simulink model "HX_Simulink_Model"  (R2024a)
settings: Solver=FixedStepAuto  StartTime=0.0  StopTime=stopTime  FixedStep=0.005  RelTol=1e-3
undefined symbols (not defined in the file or in its folder): K1_user
libraries: geometricFinDataPreCooler_WithK1TcLosses x1
settings Model: Creator=rmpel  LastModifiedBy=rmpel

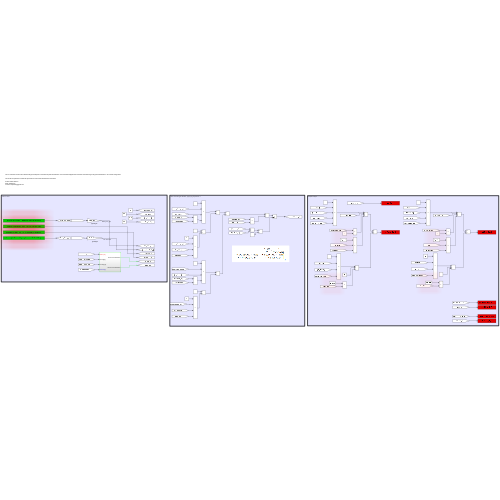
[thumbnail: Simulink's stored preview of the top-level diagram]
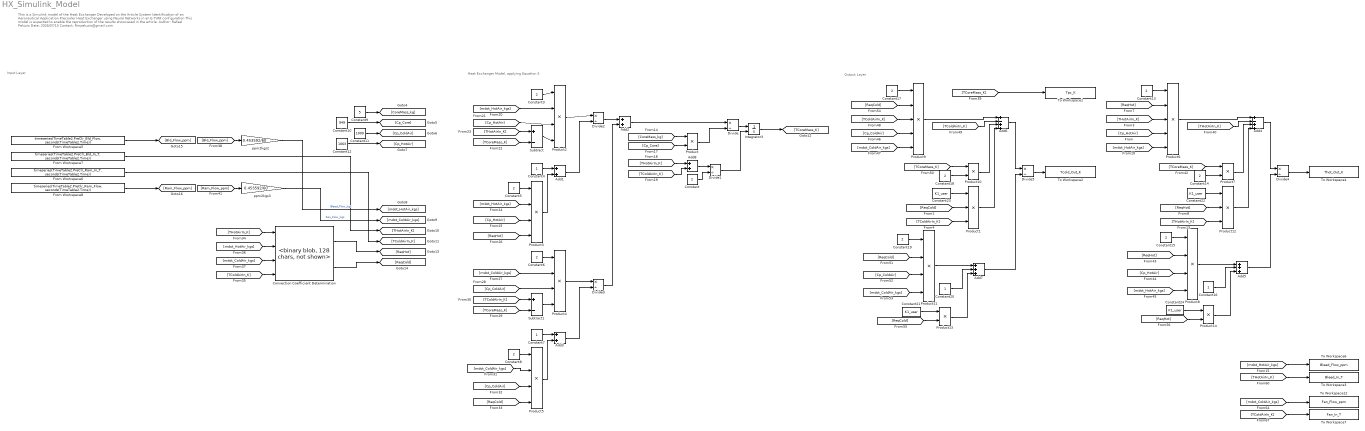
== system HX_Simulink_Model ==
  note: This is a Simulink model of the Heat Exchanger Developed on the Article System Identification of an Aeronautical Application Precooler Heat Exchanger using Neural Networks in an E-TUNI configuration
      |
      | This model is expected to enable the reproduction of the results showcased in the article.
      |
      | Author: Rafael Peluzio
      | Date: 2026/07/15
      | Contact: Rmpeluzio@gmail.com
  note: Output Layer
  note: Input Layer
  note: Heat Exchanger Model, applying Equation 3
  Add{1..3,8} (4 alike) : Sum
  Add4 : Sum  Inputs=+-++
  Add5 : Sum  Inputs=+++
  Add6 : Sum  Inputs=+-++
  Add7 : Sum  Inputs=+++
  Constant{,3,5..6,8,13..15,17..19} (11 alike) : Constant  Value=2
  Constant10 : Constant  Value=949
  Constant11 : Constant  Value=1009
  Constant12 : Constant  Value=1063
  Constant{4,7,16,20} (4 alike) : Constant
  Constant{21..24} (4 alike) : Constant  Value=K1_user
  Constant9 : Constant  Value=5
  Convection Coefficient Determination : geometricFinDataPreCooler_WithK1TcLosses/Geometric Fin Data Pre-Cooler/Temperature Dynamics/Convection Coefficient Determination  SystemSampleTime=-1  VariantActivationTime=update diagram  AllowFlexibleInterface=on  Latency=0  AutoFrameSizeCalculation=off
      link override Fin Convection//Conduction Thermal Resistance Cold Side: pitch=20/0.0254  ta=0.004*0.0254  La=0.125*0.0254  nLayers=19  layerDepth=2.75*0.0254  layerWidth=6*0.0254  layerHeight=0.231*0.0254  plateThickness=0.004*0.0254
      link override Fin Convection//Conduction Thermal Resistance Cold Side/Offset-Fin Plate-Fin Convection Coefficient Calculation/Prandtl Calculation/Specific Heat at Constant Pressure (cp) Air: Value=1.37*287/(1.37 - 1)
      link override Fin Convection//Conduction Thermal Resistance Hot Side: pitch=20/0.0254  ta=0.006*0.0254  La=0.125*0.0254  nLayers=18  layerDepth=6*0.0254  layerWidth=2.75*0.0254  layerHeight=0.181*0.0254  plateThickness=0.004*0.0254
      link override Fin Convection//Conduction Thermal Resistance Hot Side/Offset-Fin Plate-Fin Convection Coefficient Calculation/Prandtl Calculation/Specific Heat at Constant Pressure (cp) Air: Value=1.37*287/(1.37 - 1)
  Divide{,1..5} (6 alike) : Product  Inputs=*/
  From Workspace5 : FromWorkspace  VariableName=timeseries(TimeTable2.PreClr_Bld_Flow, seconds(TimeTable2.Time))
  From Workspace6 : FromWorkspace  VariableName=timeseries(TimeTable2.PreClr_Ram_In_T, seconds(TimeTable2.Time))
  From Workspace7 : FromWorkspace  VariableName=timeseries(TimeTable2.PreClr_Bld_In_T, seconds(TimeTable2.Time))
  From Workspace8 : FromWorkspace  VariableName=timeseries(TimeTable2.PreClr_Ram_Flow, seconds(TimeTable2.Time))
  Integrator3 : Integrator  InitialConditionSource=external
  Product{,7,10,13..14} (5 alike) : Product
  Product1 : Product  Inputs=3
  Product{2..5,8,11} (6 alike) : Product  Inputs=4
  Product12 : Product  Inputs=3
  Product6 : Product  Inputs=5
  Product9 : Product  Inputs=5
  Subtract : Sum  Inputs=+-
  Subtract1 : Sum  Inputs=+-
  To Workspace1 : ToWorkspace  VariableName=Tpc_K  SampleTime=-1
  To Workspace12 : ToWorkspace  VariableName=Fan_Flow_ppm  SampleTime=-1
  To Workspace2 : ToWorkspace  VariableName=Tcold_Out_K  SampleTime=-1
  To Workspace3 : ToWorkspace  VariableName=Bleed_In_T  SampleTime=-1
  To Workspace4 : ToWorkspace  VariableName=Thot_Out_K  SampleTime=-1
  To Workspace6 : ToWorkspace  VariableName=Bleed_Flow_ppm  SampleTime=-1
  To Workspace7 : ToWorkspace  VariableName=Fan_In_T  SampleTime=-1
  ppm2kgs2 : Gain  Gain=0.453592/60
  ppm2kgs3 : Gain  Gain=0.453592/60
  wires:
  Divide/1 -> Integrator3/1
  [CoreMass_kg] -> Product/1
  [Cp_Core] -> Product/2
  Product/1 -> Divide/2
  Integrator3/1 -> [TCoreMass_K]
  Constant/1 -> Divide1/2
  Add8/1 -> Divide1/1
  [THotAirIn_K] -> Add8/1
  [TColdAirIn_K] -> Add8/2
  Divide1/1 -> Integrator3/2
  [THotAirIn_K] -> Subtract/1
  [TCoreMass_K] -> Subtract/2
  Constant3/1 -> Product2/1
  [mdot_HotAir_kgs] -> Product2/2
  [Cp_HotAir] -> Product2/3
  Subtract/1 -> Product2/4
  Product2/1 -> Divide2/1
  Constant4/1 -> Add1/1
  Product3/1 -> Add1/2
  Add1/1 -> Divide2/2
  Constant5/1 -> Product3/1
  [Cp_HotAir] -> Product3/3
  [mdot_HotAir_kgs] -> Product3/2
  [ReqHot] -> Product3/4
  Divide2/1 -> Add2/1
  [ReqCold] -> Product5/4
  [Cp_ColdAir] -> Product5/3
  Constant8/1 -> Product5/1
  Add3/1 -> Divide3/2
  Product5/1 -> Add3/2
  Constant7/1 -> Add3/1
  Product4/1 -> Divide3/1
  Subtract1/1 -> Product4/4
  [Cp_ColdAir] -> Product4/3
  [mdot_ColdAir_kgs] -> Product4/2
  Constant6/1 -> Product4/1
  [TCoreMass_K] -> Subtract1/2
  [TColdAirIn_K] -> Subtract1/1
  Divide3/1 -> Add2/2
  Add2/1 -> Divide/1
  Convection Coefficient Determination/1 -> [ReqHot]
  Convection Coefficient Determination/2 -> [ReqCold]
  [mdot_ColdAir_kgs] -> Convection Coefficient Determination/3
  [TColdAirIn_K] -> Convection Coefficient Determination/4
  [mdot_HotAir_kgs] -> Convection Coefficient Determination/2
  [THotAirIn_K] -> Convection Coefficient Determination/1
  [Bld_Flow_ppm] -> ppm2kgs2/1
  From Workspace7/1 -> [THotAirIn_K]
  From Workspace6/1 -> [TColdAirIn_K]
  [Ram_Flow_ppm] -> ppm2kgs3/1
  ppm2kgs3/1 -> [mdot_ColdAir_kgs]  "Fan_Flow_kgs"
  ppm2kgs2/1 -> [mdot_HotAir_kgs]  "Bleed_Flow_kgs"
  Constant9/1 -> [CoreMass_kg]
  Constant10/1 -> [Cp_Core]
  Constant11/1 -> [Cp_ColdAir]
  Constant12/1 -> [Cp_HotAir]
  [TCoreMass_K] -> To Workspace1/1
  Constant13/1 -> Product6/1
  [ReqHot] -> Product6/2
  [THotAirIn_K] -> Product6/3
  [Cp_HotAir] -> Product6/4
  [mdot_HotAir_kgs] -> Product6/5
  [TCoreMass_K] -> Product7/1
  Constant14/1 -> Product7/2
  Product6/1 -> Add4/1
  [THotAirIn_K] -> Add4/2
  Product7/1 -> Add4/3
  Add4/1 -> Divide4/1
  [mdot_HotAir_kgs] -> Product8/4
  [Cp_HotAir] -> Product8/3
  [ReqHot] -> Product8/2
  Constant15/1 -> Product8/1
  Constant16/1 -> Add5/2
  Product8/1 -> Add5/1
  Add5/1 -> Divide4/2
  Divide4/1 -> To Workspace4/1
  Divide5/1 -> To Workspace2/1
  Add7/1 -> Divide5/2
  Product11/1 -> Add7/1
  Constant20/1 -> Add7/2
  Constant19/1 -> Product11/1
  [ReqCold] -> Product11/2
  [Cp_ColdAir] -> Product11/3
  [mdot_ColdAir_kgs] -> Product11/4
  Add6/1 -> Divide5/1
  Product10/1 -> Add6/3
  [TColdAirIn_K] -> Add6/2
  Product9/1 -> Add6/1
  Constant18/1 -> Product10/2
  [TCoreMass_K] -> Product10/1
  [mdot_ColdAir_kgs] -> Product9/5
  [Cp_ColdAir] -> Product9/4
  [TColdAirIn_K] -> Product9/3
  [ReqCold] -> Product9/2
  Constant17/1 -> Product9/1
  [TColdAirIn_K] -> Product1/3
  [ReqCold] -> Product1/2
  Constant23/1 -> Product1/1
  Product1/1 -> Add6/4
  [mdot_ColdAir_kgs] -> Product5/2
  From Workspace8/1 -> [Ram_Flow_ppm]
  From Workspace5/1 -> [Bld_Flow_ppm]
  [ReqCold] -> Product13/2
  Constant21/1 -> Product13/1
  Product13/1 -> Add7/3
  Product12/1 -> Add4/4
  [ReqHot] -> Product12/2
  [THotAirIn_K] -> Product12/3
  Constant22/1 -> Product12/1
  Constant24/1 -> Product14/1
  [ReqHot] -> Product14/2
  Product14/1 -> Add5/3
  [TColdAirIn_K] -> To Workspace7/1
  [mdot_HotAir_kgs] -> To Workspace6/1
  [mdot_ColdAir_kgs] -> To Workspace12/1
  [THotAirIn_K] -> To Workspace3/1
